simulink model "spring_measurements"  (R2014a)
settings: Solver=FixedStepDiscrete  StartTime=0.0  StopTime=inf  FixedStep=sample_time  RelTol=1e-3
values from neighbouring files (symbols this model uses):
  sample_time = 1/update_freq    (= 0.001)    [init_spring_measurements.m]
undefined symbols (not defined in the file or in its folder): A1_notch_f1, A2_notch_f1, A_lpf_accel, A_lpf_dtau, B1_lpf_accel, B1_lpf_dtau, B1_notch_f1, B2_lpf_accel, B2_lpf_dtau, B2_notch_f1, boom_mount_angle, chirp_amplitude, chirp_bias, chirp_sweep_time, control_start_time, DiscIntNeverNeededParam, ff_motor_position_back, ff_motor_position_front, hip_gravity_compensation, i_limit_lateral, j_segments, k_ff, K_notch_f1, k_sea, kd_lateral, kd_motor_position, kd_motor_velocity, kd_ratio, kd_sea_torque_flight, kd_sea_torque_stance, ki_lateral, kp_lateral, kp_motor_position, kp_motor_velocity, kp_sea_torque_flight, kp_sea_torque_stance, l_seg, lateral_torque_ramp_time, max_sagittal_loaded_torque, max_sagittal_unloaded_torque, max_torque_lateral, sagittal_torque_ramp_time, sawtooth_peak_value, sawtooth_slope, sea_control_torque_cmd_small_threshold, sea_coulomb_friction, sea_extra_moving_friction, sea_offset_friction, sea_static_friction, sine_freq, stance_flight_torque_threshold
libraries: simulink x13, dspsrcs4 x1
settings Model: BufferReuse=off  Creator=wmartin  LastModifiedBy=wmartin
settings SolverCC: EnableConcurrentExecution=on
settings DataIOCC: MaxDataPoints=1000000000  SaveFormat=StructureWithTime
settings OptimizationCC: BlockReduction=off  OptimizeBlockIOStorage=off  BufferReuse=off  GlobalBufferReuse=off  ExpressionFolding=off  ExpressionDepthLimit=2147483647  LocalBlockOutputs=off  SimCompilerOptimization=On
settings DebuggingCC: UnderspecifiedInitializationDetection=Classic  StateNameClashWarn=warning
settings HardwareCC: ProdIntDivRoundTo=Zero  ProdEndianess=LittleEndian  ProdHWDeviceType=Generic->32-bit x86 compatible
settings RTWCC: SystemTargetFile=slrt.tlc  TemplateMakefile=slrt_default_tmf  Description=Simulink Real-Time  RTWVerbose=off  ProcessScript=slrt_make_rtw_hook  RTWCompilerOptimization=On
settings SimulinkRealTimeCC: GeneratePreprocessorConditionals=Disable all  EnableShiftOperators=on  RL32LogBufSizeModifier=100000000

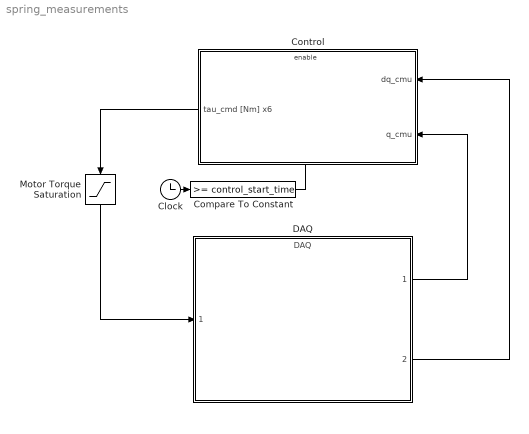
== system spring_measurements ==
  Clock : Clock
  Compare To Constant : simulink/Logic and Bit Operations/Compare To Constant  relop=>=  const=control_start_time  OutDataTypeStr=boolean
  Control : Subsystem
  DAQ : ModelReference  ModelNameDialog=DAQ  SimulationMode=Normal  ModelReferenceVersion=1.1394  CopyOfModelName=DAQ  DefaultDataLogging=on
  Motor Torque Saturation : Saturate  UpperLimit=178.5  LowerLimit=-178.5
      settings: AttributesFormatString=Top: %<UpperLimit>\nBottom: %<LowerLimit>
  wires:
  Clock/1 -> Compare To Constant/1
  Motor Torque Saturation/1 -> DAQ/1
  Compare To Constant/1 -> Control/Enable
  DAQ/1 -> Control/2(q_cmu)
  DAQ/2 -> Control/1(dq_cmu)
  Control/1(tau_cmd [Nm] x6) -> Motor Torque Saturation/1

== system spring_measurements/Control ==
  dq_cmu : Inport
  q_cmu : Inport  Port=2
  Enable : EnablePort  StatesWhenEnabling=reset
  Actuator Control : Subsystem
  Behavior Control : Subsystem
  tau_cmd [Nm] x6 : Outport  InitialOutput=[0 0 0 0 0 0]
  wires:
  q_cmu/1 -> Behavior Control/2(q_cmu), Actuator Control/2(q_cmu)
  dq_cmu/1 -> Behavior Control/1(dq_cmu), Actuator Control/3(dq_cmu)
  Actuator Control/1(tau_cmd [Nm] x6) -> tau_cmd [Nm] x6/1
  Behavior Control/1(motor_torque_cmd) -> Actuator Control/1(tau_desired [Nm] x6)

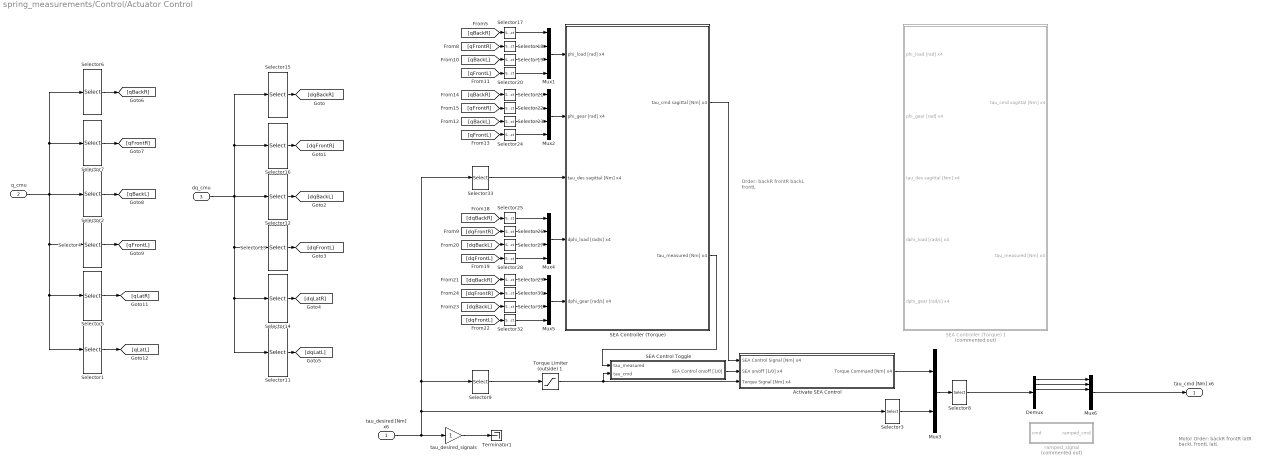
== system spring_measurements/Control/Actuator Control ==
  note: Order:
      | backR
      | frontR
      | backL
      | frontL
  note: Motor Order:
      |
      | backR
      | frontR
      | latR
      | backL
      | frontL
      | latL
  tau_desired [Nm] x6 : Inport
  q_cmu : Inport  Port=2
  dq_cmu : Inport  Port=3
  Activate SEA Control : Subsystem
  Demux : Demux  Outputs=6
  Mux{1..2,4..5} (4 alike) : Mux
  Mux3 : Mux  Inputs=2
  Mux6 : Mux  Inputs=6
  SEA Control Toggle : Subsystem
  SEA Controller (Torque) : Subsystem
  SEA Controller (Torque) 1 : Subsystem  Commented=on
  Selector1 : Selector  InputPortWidth=13  Indices=[10]
  Selector11 : Selector  InputPortWidth=13  Indices=[10]
  Selector12 : Selector  InputPortWidth=13  Indices=[5 6]
  Selector13 : Selector  InputPortWidth=13  Indices=[7 8]
  Selector14 : Selector  InputPortWidth=13  Indices=[9]
  Selector15 : Selector  InputPortWidth=13  Indices=[1 2]
  Selector16 : Selector  InputPortWidth=13  Indices=[3 4]
  Selector{17..20,25..28} (8 alike) : Selector  InputPortWidth=2  Indices=[1]
  Selector2 : Selector  InputPortWidth=13  Indices=[5 6]
  Selector{21..24,29..32} (8 alike) : Selector  InputPortWidth=2  Indices=[2]
  Selector3 : Selector  InputPortWidth=6  Indices=[3 6]
  Selector33 : Selector  InputPortWidth=6  Indices=[1 2 4 5]
  Selector4 : Selector  InputPortWidth=13  Indices=[7 8]
  Selector5 : Selector  InputPortWidth=13  Indices=[9]
  Selector6 : Selector  InputPortWidth=13  Indices=[1 2]
  Selector7 : Selector  InputPortWidth=13  Indices=[3 4]
  Selector8 : Selector  InputPortWidth=6  Indices=[1 2 5 3 4 6]
  Selector9 : Selector  InputPortWidth=6  Indices=[1 2 4 5]
  Terminator1 : Terminator
  Torque Limiter (outside) 1 : Saturate  UpperLimit=max_sagittal_unloaded_torque  LowerLimit=-max_sagittal_unloaded_torque
      settings: AttributesFormatString=Hi: %<UpperLimit>\nLo: %<LowerLimit>
  ramped_signal : Subsystem  Commented=on
  tau_desired_signals : Gain  Description=xPCTag(1)=tau_cmd_signal;
  tau_cmd [Nm] x6 : Outport  InitialOutput=[0 0 0 0 0 0]
  wires:
  Torque Limiter (outside) 1/1 -> SEA Control Toggle/2(tau_cmd), Activate SEA Control/3(Torque Signal [Nm] x4)
  SEA Controller (Torque)/1(tau_cmd sagittal [Nm] x4) -> Activate SEA Control/1(SEA Control Signal [Nm] x4)
  tau_desired [Nm] x6/1 -> tau_desired_signals/1, Selector3/1, Selector33/1, Selector9/1
  Mux6/1 -> tau_cmd [Nm] x6/1
  tau_desired_signals/1 -> Terminator1/1
  Selector5/1 -> [qLatR]
  Selector1/1 -> [qLatL]
  Selector6/1 -> [qBackR]
  Selector7/1 -> [qFrontR]
  Selector2/1 -> [qBackL]
  Selector4/1 -> [qFrontL]
  q_cmu/1 -> Selector1/1, Selector5/1, Selector4/1, Selector6/1, Selector7/1, Selector2/1
  dq_cmu/1 -> Selector12/1, Selector16/1, Selector15/1, Selector13/1, Selector14/1, Selector11/1
  Selector14/1 -> [dqLatR]
  Selector11/1 -> [dqLatL]
  Selector15/1 -> [dqBackR]
  Selector16/1 -> [dqFrontR]
  Selector12/1 -> [dqBackL]
  Selector13/1 -> [dqFrontL]
  Mux1/1 -> SEA Controller (Torque)/1(phi_load [rad] x4)
  [qBackR] -> Selector17/1
  Selector17/1 -> Mux1/1
  Selector19/1 -> Mux1/3
  Selector18/1 -> Mux1/2
  Selector20/1 -> Mux1/4
  [qFrontR] -> Selector18/1
  [qBackL] -> Selector19/1
  [qFrontL] -> Selector20/1
  Mux2/1 -> SEA Controller (Torque)/2(phi_gear [rad] x4)
  [qBackR] -> Selector21/1
  Selector21/1 -> Mux2/1
  Selector23/1 -> Mux2/3
  Selector22/1 -> Mux2/2
  Selector24/1 -> Mux2/4
  [qFrontR] -> Selector22/1
  [qBackL] -> Selector23/1
  [qFrontL] -> Selector24/1
  Mux4/1 -> SEA Controller (Torque)/4(dphi_load [rad/s] x4)
  [dqBackR] -> Selector25/1
  Selector25/1 -> Mux4/1
  Selector27/1 -> Mux4/3
  Selector26/1 -> Mux4/2
  Selector28/1 -> Mux4/4
  [dqFrontR] -> Selector26/1
  [dqBackL] -> Selector27/1
  [dqFrontL] -> Selector28/1
  Mux5/1 -> SEA Controller (Torque)/5(dphi_gear [rad/s] x4)
  [dqBackR] -> Selector29/1
  Selector29/1 -> Mux5/1
  Selector31/1 -> Mux5/3
  Selector30/1 -> Mux5/2
  Selector32/1 -> Mux5/4
  [dqFrontR] -> Selector30/1
  [dqBackL] -> Selector31/1
  [dqFrontL] -> Selector32/1
  Selector33/1 -> SEA Controller (Torque)/3(tau_des sagittal [Nm] x4)
  Selector3/1 -> Mux3/2
  Mux3/1 -> Selector8/1
  Selector8/1 -> Demux/1
  Demux/3 -> Mux6/3
  Demux/1 -> Mux6/1
  Demux/2 -> Mux6/2
  Selector9/1 -> Torque Limiter (outside) 1/1
  SEA Controller (Torque)/2(tau_measured [Nm] x4) -> SEA Control Toggle/1(tau_measured)
  SEA Control Toggle/1(SEA Control on/off [1/0]) -> Activate SEA Control/2("SEA on/off [1/0] x4 ")
  Activate SEA Control/1(Torque Command [Nm] x4) -> Mux3/1

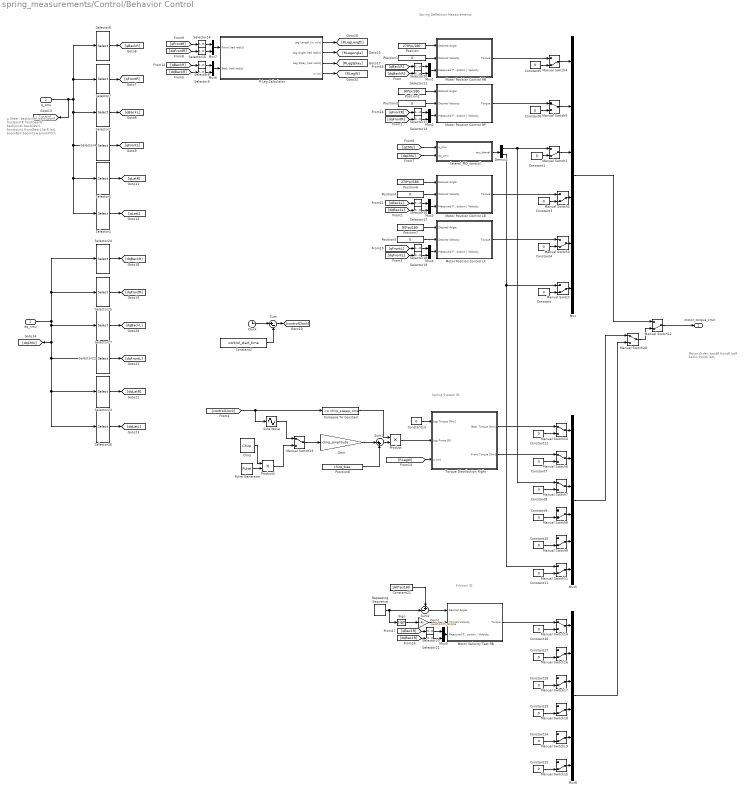
== system spring_measurements/Control/Behavior Control ==
  note: Spring Deflection Measurements
  note: q Order:
      |
      | backJointR
      | backGearR
      | frontJointR
      | frontGearR
      |
      | backJointL
      | backGearL
      | frontJointL
      | frontGearL
      |
      | latR
      | latL
      |
      | boomRoll
      | boomYaw
      | boomPitch
  note: Motor Order:
      |
      | backR
      | frontR
      | latR
      | backL
      | frontL
      | latL
  note: Spring System ID
  note: Friction ID
  dq_cmu : Inport
  q_cmu : Inport  Port=2
  Chirp : dspsrcs4/Chirp  sweep=Quadratic  mode=Unidirectional  f0=chirp_min_freq  f1=chirp_max_freq  t1=chirp_sweep_time  Tsweep=chirp_sweep_time  phase=0  Ts=sample_time  spf=1  datatype=Double
  Clock : Clock
  Compare To Constant : simulink/Logic and Bit Operations/Compare To Constant  relop=<=  const=chirp_sweep_time  OutDataTypeStr=uint8
  Constant{,1,3..19} (19 alike) : Constant  Value=0
  Constant2 : Constant  Value=control_start_time
  Constant21 : Constant  Value=160*pi/180
  Demux2 : Demux  Outputs=2
  Gain : Gain  Gain=chirp_amplitude
  Gain1 : Gain  Gain=-sawtooth_slope
  Manual Switch{,1..4,8..9,11..12,15..19} (14 alike) : ManualSwitch  CurrentSetting=0
  Manual Switch{5..7,10,13..14,20} (7 alike) : ManualSwitch
  Motor Position Control LB : Subsystem
  Motor Position Control LF : Subsystem
  Motor Position Control RB : Subsystem
  Motor Position Control RF : Subsystem
  Motor Velocity Test RB : Subsystem
  Mux : Mux  Inputs=6
  Mux{1..4,6..7,9} (7 alike) : Mux  Inputs=2
  Mux5 : Mux  Inputs=6
  Mux8 : Mux  Inputs=6
  Position : Constant  Value=270*pi/180
  Position{1,3..5} (4 alike) : Constant  Value=0
  Position2 : Constant  Value=90*pi/180
  Position6 : Constant  Value=270*pi/180
  Position7 : Constant  Value=90*pi/180
  Position8 : Constant  Value=chirp_bias
  Product : Product
  Product1 : Product
  Pulse Generator : DiscretePulseGenerator  PulseType=Time based  Period=10  PulseWidth=50
  R Leg Calculator : Subsystem
  Repeating Sequence : simulink/Sources/Repeating Sequence  rep_seq_t=sawtooth_time_values  rep_seq_y=[0 sawtooth_peak_value 0]
  Selector1 : Selector  InputPortWidth=13  Indices=[10]
  Selector{10..13,16..21} (10 alike) : Selector  InputPortWidth=2  Indices=[2]
  Selector{8..9,14..15} (4 alike) : Selector  InputPortWidth=2  Indices=[1]
  Selector2 : Selector  InputPortWidth=13  Indices=[5 6]
  Selector22 : Selector  InputPortWidth=13  Indices=[7 8]
  Selector23 : Selector  InputPortWidth=13  Indices=[9]
  Selector24 : Selector  InputPortWidth=13  Indices=[1 2]
  Selector25 : Selector  InputPortWidth=13  Indices=[3 4]
  Selector26 : Selector  InputPortWidth=13  Indices=[10]
  Selector27 : Selector  InputPortWidth=13  Indices=[5 6]
  Selector4 : Selector  InputPortWidth=13  Indices=[7 8]
  Selector5 : Selector  InputPortWidth=13  Indices=[9]
  Selector6 : Selector  InputPortWidth=13  Indices=[1 2]
  Selector7 : Selector  InputPortWidth=13  Indices=[3 4]
  Sign : Signum
  Sine Wave : Sin  TimeSource=Use external signal  Frequency=sine_freq  SampleTime=0
  Sum : Sum  Inputs=|+-
  Sum1 : Sum  Inputs=|++
  Sum2 : Sum  Inputs=+-|
  Torque Distribution Right : Subsystem
  lateral_PID_control : Subsystem
  motor_torque_cmd : Outport  OutputWhenDisabled=reset  InitialOutput=[0 0 0 0 0 0]
  wires:
  Mux/1 -> Manual Switch12/1
  Demux2/1 -> Manual Switch7/1, Manual Switch1/1
  Demux2/2 -> Manual Switch11/1, Manual Switch/1
  Manual Switch1/1 -> Mux/3
  Manual Switch/1 -> Mux/6
  Constant/1 -> Manual Switch/2
  Constant1/1 -> Manual Switch1/2
  Clock/1 -> Sum/1
  Constant2/1 -> Sum/2
  Selector5/1 -> [qLatR]
  Selector1/1 -> [qLatL]
  Sum/1 -> [controlClock]
  Selector12/1 -> Mux2/1
  Selector16/1 -> Mux3/1
  Selector18/1 -> Mux4/1
  [qCMU] -> lateral_PID_control/1(q_cmu)
  [dqCMU] -> lateral_PID_control/2(dq_cmu)
  lateral_PID_control/1(tau_lateral) -> Demux2/1
  Constant3/1 -> Manual Switch2/2
  Constant4/1 -> Manual Switch3/2
  Manual Switch3/1 -> Mux/5
  Manual Switch2/1 -> Mux/4
  Motor Position Control RB/1(Torque) -> Manual Switch4/1
  Constant5/1 -> Manual Switch4/2
  Constant6/1 -> Manual Switch5/2
  Manual Switch4/1 -> Mux/1
  Manual Switch5/1 -> Mux/2
  Position/1 -> Motor Position Control RB/1(Desired Angle)
  Position1/1 -> Motor Position Control RB/2(Desired Velocity)
  Mux1/1 -> Motor Position Control RB/3(Measured Position / Velocity)
  Selector11/1 -> Mux1/2
  Selector10/1 -> Mux1/1
  Motor Position Control RF/1(Torque) -> Manual Switch5/1
  Mux2/1 -> Motor Position Control RF/3(Measured Position / Velocity)
  Selector13/1 -> Mux2/2
  Position3/1 -> Motor Position Control RF/2(Desired Velocity)
  Position2/1 -> Motor Position Control RF/1(Desired Angle)
  Motor Position Control LB/1(Torque) -> Manual Switch2/1
  Motor Position Control LF/1(Torque) -> Manual Switch3/1
  Mux3/1 -> Motor Position Control LB/3(Measured Position / Velocity)
  Mux4/1 -> Motor Position Control LF/3(Measured Position / Velocity)
  Selector17/1 -> Mux3/2
  Selector19/1 -> Mux4/2
  Position4/1 -> Motor Position Control LB/2(Desired Velocity)
  Position5/1 -> Motor Position Control LF/2(Desired Velocity)
  Position6/1 -> Motor Position Control LB/1(Desired Angle)
  Position7/1 -> Motor Position Control LF/1(Desired Angle)
  Constant12/1 -> Manual Switch10/2
  Constant7/1 -> Manual Switch6/2
  Manual Switch6/1 -> Mux5/2
  Constant8/1 -> Manual Switch7/2
  Manual Switch7/1 -> Mux5/3
  Constant9/1 -> Manual Switch8/2
  Constant10/1 -> Manual Switch9/2
  Constant11/1 -> Manual Switch11/2
  Manual Switch11/1 -> Mux5/6
  Manual Switch9/1 -> Mux5/5
  Manual Switch12/1 -> motor_torque_cmd/1
  Mux5/1 -> Manual Switch20/1
  Manual Switch13/1 -> Gain/1
  [controlClock] -> Sine Wave/1, Compare To Constant/1
  Compare To Constant/1 -> Product/1
  Sum1/1 -> Product/2
  Gain/1 -> Sum1/1
  Position8/1 -> Sum1/2
  Manual Switch10/1 -> Mux5/1
  Manual Switch8/1 -> Mux5/4
  Chirp/1 -> Product1/1
  Sine Wave/1 -> Manual Switch13/1
  Pulse Generator/1 -> Product1/2
  Product1/1 -> Manual Switch13/2
  Product/1 -> Torque Distribution Right/2(Leg Force [N])
  Torque Distribution Right/1(Back Torque [Nm]) -> Manual Switch10/1
  Torque Distribution Right/2(Front Torque [Nm]) -> Manual Switch6/1
  Constant13/1 -> Torque Distribution Right/1(Leg Torque [Nm])
  Mux7/1 -> R Leg Calculator/1(Front [rad rad/s])
  Mux6/1 -> R Leg Calculator/2(Back [rad rad/s])
  R Leg Calculator/1("Leg Length [m m/s] ") -> [RLegLength]
  R Leg Calculator/2(Leg Angle [rad rad/s]) -> [RLegAngle]
  R Leg Calculator/3(Leg Splay [rad rad/s]) -> [RLegSplay]
  Selector14/1 -> Mux7/1
  Selector15/1 -> Mux7/2
  Selector9/1 -> Mux6/2
  Selector8/1 -> Mux6/1
  R Leg Calculator/4(w [m]) -> [RLegW]
  [RLegW] -> Torque Distribution Right/3(w [m])
  Constant16/1 -> Manual Switch14/2
  Constant17/1 -> Manual Switch16/2
  Manual Switch16/1 -> Mux8/2
  Constant18/1 -> Manual Switch17/2
  Manual Switch17/1 -> Mux8/3
  Constant19/1 -> Manual Switch18/2
  Constant14/1 -> Manual Switch19/2
  Constant15/1 -> Manual Switch15/2
  Manual Switch15/1 -> Mux8/6
  Manual Switch19/1 -> Mux8/5
  Mux8/1 -> Manual Switch20/2
  Manual Switch14/1 -> Mux8/1
  Manual Switch18/1 -> Mux8/4
  Motor Velocity Test RB/1(Torque) -> Manual Switch14/1
  q_cmu/1 -> [qCMU], Selector6/1, Selector7/1, Selector2/1, Selector4/1, Selector1/1, Selector5/1
  Selector4/1 -> [qFrontL]
  Selector2/1 -> [qBackL]
  Selector7/1 -> [qFrontR]
  Selector6/1 -> [qBackR]
  [dqBackR] -> Selector9/1
  [qBackR] -> Selector8/1
  [dqFrontR] -> Selector15/1
  [qFrontR] -> Selector14/1
  [qBackR] -> Selector10/1
  [dqBackR] -> Selector11/1
  [qFrontR] -> Selector12/1
  [dqFrontR] -> Selector13/1
  [qFrontL] -> Selector18/1
  [dqFrontL] -> Selector19/1
  [dqBackL] -> Selector17/1
  [qBackL] -> Selector16/1
  [qBackR] -> Selector20/1
  [dqBackR] -> Selector21/1
  Selector26/1 -> [dqLatL]
  Selector23/1 -> [dqLatR]
  Selector24/1 -> [dqBackR]
  Selector25/1 -> [dqFrontR]
  Selector27/1 -> [dqBackL]
  Selector22/1 -> [dqFrontL]
  dq_cmu/1 -> Selector27/1, Selector26/1, Selector23/1, Selector22/1, [dqCMU], Selector24/1, Selector25/1
  Repeating Sequence/1 -> Sign/1, Sum2/2
  Mux9/1 -> Motor Velocity Test RB/3(Measured Position / Velocity)
  Selector21/1 -> Mux9/2
  Selector20/1 -> Mux9/1
  Sign/1 -> Gain1/1
  Gain1/1 -> Motor Velocity Test RB/2(Desired Velocity)
  Sum2/1 -> Motor Velocity Test RB/1(Desired Angle)
  Constant21/1 -> Sum2/1
  Manual Switch20/1 -> Manual Switch12/2

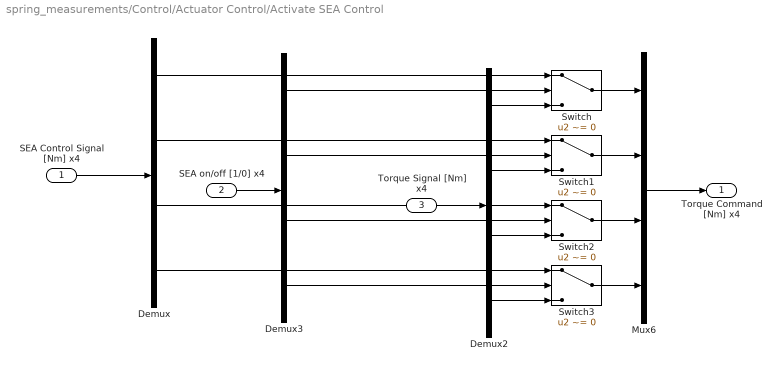
== system spring_measurements/Control/Actuator Control/Activate SEA Control ==
  SEA Control Signal [Nm] x4 : Inport
  "SEA on/off [1/0] x4 " : Inport  Port=2
  Torque Signal [Nm] x4 : Inport  Port=3
  Demux : Demux
  Demux2 : Demux
  Demux3 : Demux
  Mux6 : Mux
  Switch{,1..3} (4 alike) : Switch  Criteria=u2 ~= 0
  Torque Command [Nm] x4 : Outport
  wires:
  Torque Signal [Nm] x4/1 -> Demux2/1
  "SEA on/off [1/0] x4 "/1 -> Demux3/1
  SEA Control Signal [Nm] x4/1 -> Demux/1
  Demux2/3 -> Switch2/3
  Demux/2 -> Switch1/1
  Demux3/4 -> Switch3/2
  Demux2/4 -> Switch3/3
  Demux/4 -> Switch3/1
  Switch2/1 -> Mux6/3
  Demux/3 -> Switch2/1
  Demux3/2 -> Switch1/2
  Demux3/3 -> Switch2/2
  Mux6/1 -> Torque Command [Nm] x4/1
  Demux3/1 -> Switch/2
  Switch3/1 -> Mux6/4
  Switch1/1 -> Mux6/2
  Switch/1 -> Mux6/1
  Demux/1 -> Switch/1
  Demux2/1 -> Switch/3
  Demux2/2 -> Switch1/3

== system spring_measurements/Control/Actuator Control/SEA Control Toggle ==
  tau_measured : Inport
  tau_cmd : Inport  Port=2
  Abs : Abs
  Abs1 : Abs
  But Commanding a Small Torque? : simulink/Logic and Bit Operations/Compare To Constant  relop=<  const=sea_control_torque_cmd_small_threshold  OutDataTypeStr=boolean
  Logical Operator1 : Logic  AllPortsSameDT=off  OutDataTypeStr=boolean
  Logical Operator2 : Logic  Operator=NOT  AllPortsSameDT=off  OutDataTypeStr=boolean
  Measuring a Large Torque? (High Gains) : simulink/Logic and Bit Operations/Compare To Constant  relop=>=  const=stance_flight_torque_threshold  OutDataTypeStr=boolean
  SEA Control on/off [1/0] : Outport
  wires:
  Abs1/1 -> Measuring a Large Torque? (High Gains)/1
  Measuring a Large Torque? (High Gains)/1 -> Logical Operator1/1
  tau_measured/1 -> Abs1/1
  Abs/1 -> But Commanding a Small Torque?/1
  tau_cmd/1 -> Abs/1
  Logical Operator1/1 -> Logical Operator2/1
  But Commanding a Small Torque?/1 -> Logical Operator1/2
  Logical Operator2/1 -> SEA Control on/off [1/0]/1

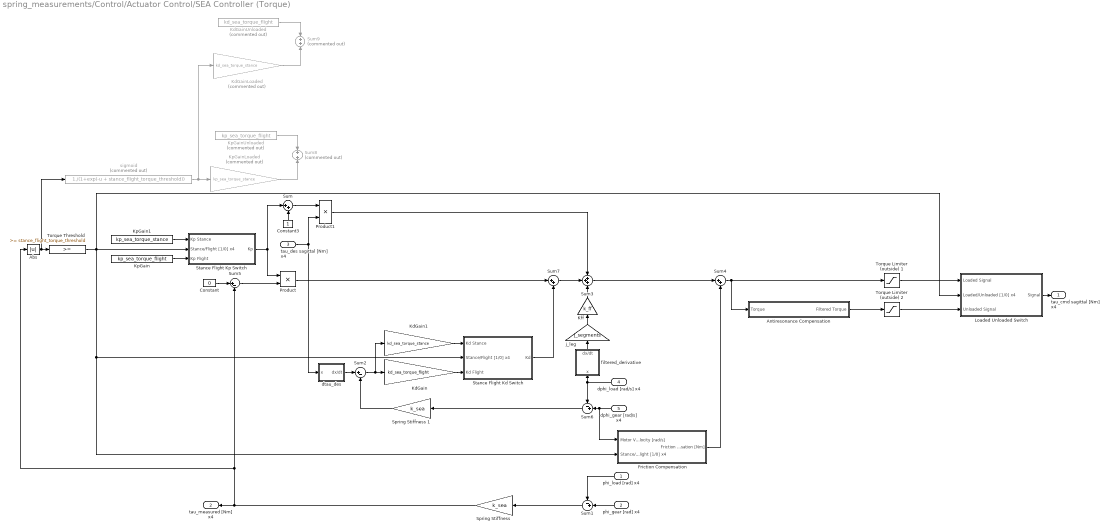
== system spring_measurements/Control/Actuator Control/SEA Controller (Torque) ==
  phi_load [rad] x4 : Inport
  phi_gear [rad] x4 : Inport  Port=2
  tau_des sagittal [Nm] x4 : Inport  Port=3
  dphi_load [rad/s] x4 : Inport  Port=4
  dphi_gear [rad/s] x4 : Inport  Port=5
  Abs : Abs
  Antiresonance Compensation : Subsystem
  Constant : Constant  Value=0
  Constant3 : Constant
  Friction Compensation : Subsystem
  KdGain : Gain  Description=xPCTag(1)=kd_sea_torque;  Gain=kd_sea_torque_flight
  KdGain1 : Gain  Description=xPCTag(1)=kd_sea_torque;  Gain=kd_sea_torque_stance
  KdGainLoaded : Gain  Description=xPCTag(1)=kd_sea_torque;  Commented=on  Gain=kd_sea_torque_stance
  KdGainUnloaded : Constant  Commented=on  Value=kd_sea_torque_flight  SampleTime=sample_time
  Kff : Gain  Gain=k_ff
  KpGain : Constant  Value=kp_sea_torque_flight  SampleTime=sample_time
  KpGain1 : Constant  Value=kp_sea_torque_stance  SampleTime=sample_time
  KpGainLoaded : Gain  Description=xPCTag(1)=kd_sea_torque;  Commented=on  Gain=kp_sea_torque_stance
  KpGainUnloaded : Constant  Commented=on  Value=kp_sea_torque_flight  SampleTime=sample_time
  Loaded Unloaded Switch : Subsystem
  Product : Product  SampleTime=sample_time  RndMeth=Zero
  Product1 : Product  RndMeth=Zero
  Spring Stiffness : Gain  Gain=k_sea
  Spring Stiffness 1 : Gain  Gain=k_sea
  Stance Flight Kd Switch : Subsystem
  Stance Flight Kp Switch : Subsystem
  Sum : Sum  Inputs=|++  SampleTime=sample_time
  Sum1 : Sum  Inputs=-+|
  Sum2 : Sum  Inputs=|+-
  Sum3 : Sum  Inputs=+++
  Sum4 : Sum  Inputs=|++
  Sum5 : Sum  Inputs=|+-
  Sum6 : Sum  Inputs=-+|
  Sum7 : Sum  Inputs=|++
  Sum8 : Sum  Commented=on  Inputs=+|+  SampleTime=sample_time
  Sum9 : Sum  Commented=on  Inputs=+|+  SampleTime=sample_time
  Torque Limiter (outside) 1 : Saturate  UpperLimit=max_sagittal_loaded_torque  LowerLimit=-max_sagittal_loaded_torque
      settings: AttributesFormatString=Hi: %<UpperLimit>\nLo: %<LowerLimit>
  Torque Limiter (outside) 2 : Saturate  UpperLimit=max_sagittal_unloaded_torque  LowerLimit=-max_sagittal_unloaded_torque
      settings: AttributesFormatString=Hi: %<UpperLimit>\nLo: %<LowerLimit>
  Torque Threshold : simulink/Logic and Bit Operations/Compare To Constant  relop=>=  const=stance_flight_torque_threshold  OutDataTypeStr=boolean
  dtau_des : Subsystem
  filtered_derivative : Subsystem
  j_leg : Gain  Description=xPCTag(1)=kd_sea_torque;  Gain=j_segments
  sigmoid : Fcn  Commented=on  Expr=1./(1+exp(-u + stance_flight_torque_threshold))
  tau_cmd sagittal [Nm] x4 : Outport
  tau_measured [Nm] x4 : Outport  Port=2
  wires:
  KdGainLoaded/1 -> Sum9/2
  KdGainUnloaded/1 -> Sum9/1
  KpGainLoaded/1 -> Sum8/2
  KpGainUnloaded/1 -> Sum8/1
  sigmoid/1 -> KpGainLoaded/1, KdGainLoaded/1
  Loaded Unloaded Switch/1(Signal) -> tau_cmd sagittal [Nm] x4/1
  Torque Limiter (outside) 2/1 -> Loaded Unloaded Switch/3(Unloaded Signal)
  Friction Compensation/1(Friction Compensation [Nm]) -> Sum4/2
  tau_des sagittal [Nm] x4/1 -> Product1/2, dtau_des/1(x)
  Kff/1 -> Sum3/3
  Torque Limiter (outside) 1/1 -> Loaded Unloaded Switch/1(Loaded Signal)
  j_leg/1 -> Kff/1
  filtered_derivative/1(dx/dt) -> j_leg/1
  Sum/1 -> Product1/1
  Constant3/1 -> Sum/2
  KdGain/1 -> Stance Flight Kd Switch/3(Kd Flight)
  Product/1 -> Sum7/1
  Sum5/1 -> Product/2
  Sum2/1 -> KdGain1/1, KdGain/1
  dphi_gear [rad/s] x4/1 -> Friction Compensation/1(Motor Velocity [rad/s]), Sum6/2
  dphi_load [rad/s] x4/1 -> filtered_derivative/1(x), Sum6/1
  Spring Stiffness 1/1 -> Sum2/2
  Sum6/1 -> Spring Stiffness 1/1
  dtau_des/1(dx/dt) -> Sum2/1
  Constant/1 -> Sum5/1
  phi_gear [rad] x4/1 -> Sum1/2
  phi_load [rad] x4/1 -> Sum1/1
  Sum1/1 -> Spring Stiffness/1
  KpGain1/1 -> Stance Flight Kp Switch/1(Kp Stance)
  Torque Threshold/1 -> Friction Compensation/2(Stance/Flight [1/0] x4), Stance Flight Kd Switch/2(Stance/Flight [1/0] x4), Stance Flight Kp Switch/2(Stance/Flight [1/0] x4), Loaded Unloaded Switch/2(Loaded/Unloaded [1/0] x4)
  KpGain/1 -> Stance Flight Kp Switch/3(Kp Flight)
  KdGain1/1 -> Stance Flight Kd Switch/1(Kd Stance)
  Spring Stiffness/1 -> Sum5/2, Abs/1, tau_measured [Nm] x4/1
  Stance Flight Kp Switch/1(Kp) -> Sum/1, Product/1
  Abs/1 -> Torque Threshold/1, sigmoid/1
  Stance Flight Kd Switch/1(Kd) -> Sum7/2
  Sum4/1 -> Torque Limiter (outside) 1/1, Antiresonance Compensation/1(Torque)
  Product1/1 -> Sum3/1
  Sum7/1 -> Sum3/2
  Sum3/1 -> Sum4/1
  Antiresonance Compensation/1(Filtered Torque) -> Torque Limiter (outside) 2/1

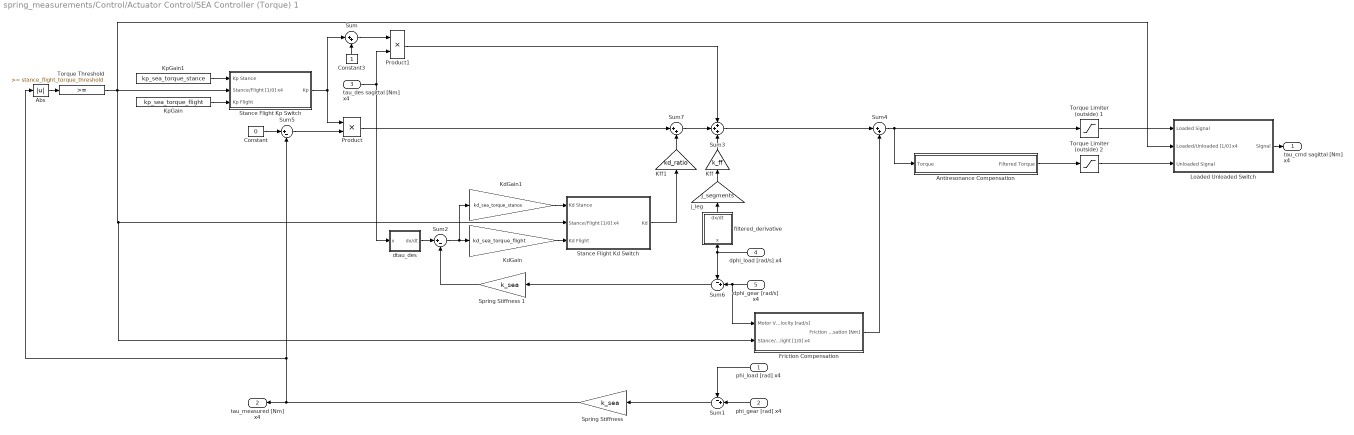
== system spring_measurements/Control/Actuator Control/SEA Controller (Torque) 1 ==
  phi_load [rad] x4 : Inport
  phi_gear [rad] x4 : Inport  Port=2
  tau_des sagittal [Nm] x4 : Inport  Port=3
  dphi_load [rad/s] x4 : Inport  Port=4
  dphi_gear [rad/s] x4 : Inport  Port=5
  Abs : Abs
  Antiresonance Compensation : Subsystem
  Constant : Constant  Value=0
  Constant3 : Constant
  Friction Compensation : Subsystem
  KdGain : Gain  Description=xPCTag(1)=kd_sea_torque;  Gain=kd_sea_torque_flight
  KdGain1 : Gain  Description=xPCTag(1)=kd_sea_torque;  Gain=kd_sea_torque_stance
  Kff : Gain  Gain=k_ff
  Kff1 : Gain  Gain=kd_ratio
  KpGain : Constant  Value=kp_sea_torque_flight  SampleTime=sample_time
  KpGain1 : Constant  Value=kp_sea_torque_stance  SampleTime=sample_time
  Loaded Unloaded Switch : Subsystem
  Product : Product  SampleTime=sample_time  RndMeth=Zero
  Product1 : Product  RndMeth=Zero
  Spring Stiffness : Gain  Gain=k_sea
  Spring Stiffness 1 : Gain  Gain=k_sea
  Stance Flight Kd Switch : Subsystem
  Stance Flight Kp Switch : Subsystem
  Sum : Sum  Inputs=|++  SampleTime=sample_time
  Sum1 : Sum  Inputs=-+|
  Sum2 : Sum  Inputs=|+-
  Sum3 : Sum  Inputs=+++
  Sum4 : Sum  Inputs=|++
  Sum5 : Sum  Inputs=|+-
  Sum6 : Sum  Inputs=-+|
  Sum7 : Sum  Inputs=|++
  Torque Limiter (outside) 1 : Saturate  UpperLimit=max_sagittal_loaded_torque  LowerLimit=-max_sagittal_loaded_torque
      settings: AttributesFormatString=Hi: %<UpperLimit>\nLo: %<LowerLimit>
  Torque Limiter (outside) 2 : Saturate  UpperLimit=max_sagittal_unloaded_torque  LowerLimit=-max_sagittal_unloaded_torque
      settings: AttributesFormatString=Hi: %<UpperLimit>\nLo: %<LowerLimit>
  Torque Threshold : simulink/Logic and Bit Operations/Compare To Constant  relop=>=  const=stance_flight_torque_threshold  OutDataTypeStr=boolean
  dtau_des : Subsystem
  filtered_derivative : Subsystem
  j_leg : Gain  Description=xPCTag(1)=kd_sea_torque;  Gain=j_segments
  tau_cmd sagittal [Nm] x4 : Outport
  tau_measured [Nm] x4 : Outport  Port=2
  wires:
  Loaded Unloaded Switch/1(Signal) -> tau_cmd sagittal [Nm] x4/1
  Torque Limiter (outside) 2/1 -> Loaded Unloaded Switch/3(Unloaded Signal)
  Friction Compensation/1(Friction Compensation [Nm]) -> Sum4/2
  tau_des sagittal [Nm] x4/1 -> Product1/2, dtau_des/1(x)
  Stance Flight Kd Switch/1(Kd) -> Kff1/1
  Kff/1 -> Sum3/3
  Torque Limiter (outside) 1/1 -> Loaded Unloaded Switch/1(Loaded Signal)
  j_leg/1 -> Kff/1
  filtered_derivative/1(dx/dt) -> j_leg/1
  Sum/1 -> Product1/1
  Constant3/1 -> Sum/2
  KdGain/1 -> Stance Flight Kd Switch/3(Kd Flight)
  Product/1 -> Sum7/1
  Sum5/1 -> Product/2
  Sum2/1 -> KdGain1/1, KdGain/1
  dphi_gear [rad/s] x4/1 -> Friction Compensation/1(Motor Velocity [rad/s]), Sum6/2
  dphi_load [rad/s] x4/1 -> filtered_derivative/1(x), Sum6/1
  Spring Stiffness 1/1 -> Sum2/2
  Sum6/1 -> Spring Stiffness 1/1
  dtau_des/1(dx/dt) -> Sum2/1
  Constant/1 -> Sum5/1
  phi_gear [rad] x4/1 -> Sum1/2
  phi_load [rad] x4/1 -> Sum1/1
  Sum1/1 -> Spring Stiffness/1
  KpGain1/1 -> Stance Flight Kp Switch/1(Kp Stance)
  Torque Threshold/1 -> Friction Compensation/2(Stance/Flight [1/0] x4), Stance Flight Kd Switch/2(Stance/Flight [1/0] x4), Stance Flight Kp Switch/2(Stance/Flight [1/0] x4), Loaded Unloaded Switch/2(Loaded/Unloaded [1/0] x4)
  KpGain/1 -> Stance Flight Kp Switch/3(Kp Flight)
  KdGain1/1 -> Stance Flight Kd Switch/1(Kd Stance)
  Spring Stiffness/1 -> Sum5/2, Abs/1, tau_measured [Nm] x4/1
  Stance Flight Kp Switch/1(Kp) -> Sum/1, Product/1
  Abs/1 -> Torque Threshold/1
  Kff1/1 -> Sum7/2
  Sum4/1 -> Torque Limiter (outside) 1/1, Antiresonance Compensation/1(Torque)
  Product1/1 -> Sum3/1
  Sum7/1 -> Sum3/2
  Sum3/1 -> Sum4/1
  Antiresonance Compensation/1(Filtered Torque) -> Torque Limiter (outside) 2/1

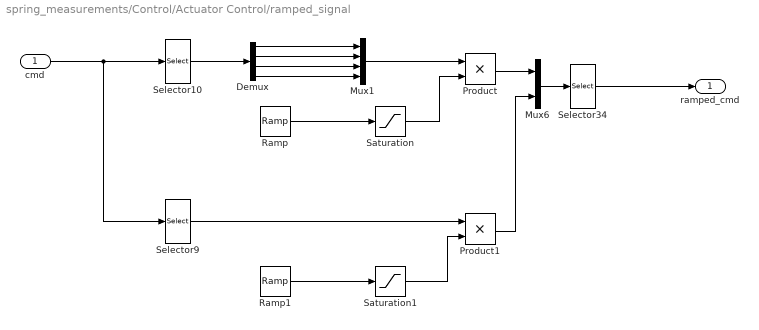
== system spring_measurements/Control/Actuator Control/ramped_signal ==
  cmd : Inport
  Demux : Demux
  Mux1 : Mux
  Mux6 : Mux  Inputs=2
  Product : Product  RndMeth=Zero
  Product1 : Product  RndMeth=Zero
  Ramp : simulink/Sources/Ramp  slope=1/sagittal_torque_ramp_time  start=sagittal_starting_time  X0=0
      settings: AttributesFormatString=Start: %<start>\nSlope: %<slope>
  Ramp1 : simulink/Sources/Ramp  slope=1/lateral_torque_ramp_time  start=control_start_time  X0=0
      settings: AttributesFormatString=Start: %<start>\nSlope: %<slope>
  Saturation : Saturate  UpperLimit=1  LowerLimit=0
      settings: AttributesFormatString=Hi: %<UpperLimit>\nLo: %<LowerLimit>
  Saturation1 : Saturate  UpperLimit=1  LowerLimit=0
      settings: AttributesFormatString=Hi: %<UpperLimit>\nLo: %<LowerLimit>
  Selector10 : Selector  InputPortWidth=6  Indices=[1 2 4 5]
  Selector34 : Selector  InputPortWidth=6  Indices=[1 2 5 3 4 6]
  Selector9 : Selector  InputPortWidth=6  Indices=[3 6]
  ramped_cmd : Outport
  wires:
  Demux/3 -> Mux1/3
  Demux/4 -> Mux1/4
  Mux1/1 -> Product/1
  Demux/2 -> Mux1/2
  Demux/1 -> Mux1/1
  Mux6/1 -> Selector34/1
  Selector10/1 -> Demux/1
  Selector34/1 -> ramped_cmd/1
  Product1/1 -> Mux6/2
  cmd/1 -> Selector9/1, Selector10/1
  Product/1 -> Mux6/1
  Ramp/1 -> Saturation/1
  Saturation/1 -> Product/2
  Ramp1/1 -> Saturation1/1
  Saturation1/1 -> Product1/2
  Selector9/1 -> Product1/1

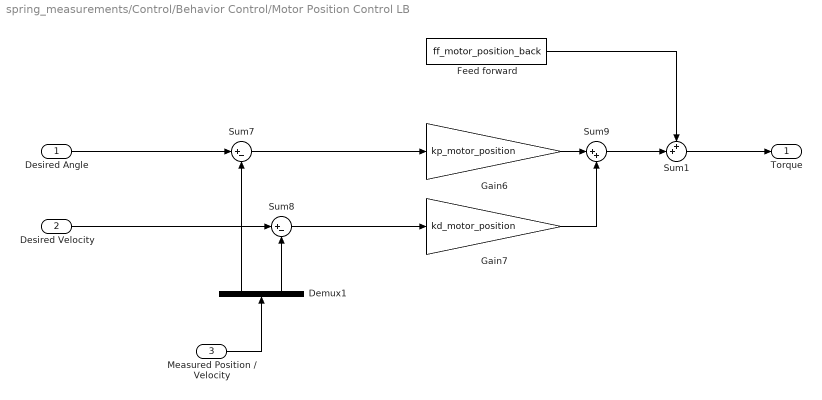
== system spring_measurements/Control/Behavior Control/Motor Position Control LB ==
  Desired Angle : Inport
  Desired Velocity : Inport  Port=2
  Measured Position / Velocity : Inport  Port=3
  Demux1 : Demux  Outputs=2
  Feed forward : Constant  Value=ff_motor_position_back
  Gain6 : Gain  Gain=kp_motor_position
  Gain7 : Gain  Gain=kd_motor_position
  Sum1 : Sum  Inputs=++|
  Sum7 : Sum  Inputs=|+-
  Sum8 : Sum  Inputs=|+-
  Sum9 : Sum  Inputs=|++
  Torque : Outport
  wires:
  Sum7/1 -> Gain6/1
  Demux1/1 -> Sum7/2
  Sum9/1 -> Sum1/2
  Desired Velocity/1 -> Sum8/1
  Sum8/1 -> Gain7/1
  Desired Angle/1 -> Sum7/1
  Demux1/2 -> Sum8/2
  Measured Position / Velocity/1 -> Demux1/1
  Gain7/1 -> Sum9/2
  Gain6/1 -> Sum9/1
  Feed forward/1 -> Sum1/1
  Sum1/1 -> Torque/1

== system spring_measurements/Control/Behavior Control/Motor Position Control LF ==
  Desired Angle : Inport
  Desired Velocity : Inport  Port=2
  Measured Position / Velocity : Inport  Port=3
  Demux1 : Demux  Outputs=2
  Feed forward : Constant  Value=ff_motor_position_front
  Gain6 : Gain  Gain=kp_motor_position
  Gain7 : Gain  Gain=kd_motor_position
  Sum1 : Sum  Inputs=++|
  Sum7 : Sum  Inputs=|+-
  Sum8 : Sum  Inputs=|+-
  Sum9 : Sum  Inputs=|++
  Torque : Outport
  wires:
  Sum1/1 -> Torque/1
  Feed forward/1 -> Sum1/1
  Gain6/1 -> Sum9/1
  Gain7/1 -> Sum9/2
  Measured Position / Velocity/1 -> Demux1/1
  Demux1/2 -> Sum8/2
  Desired Angle/1 -> Sum7/1
  Sum8/1 -> Gain7/1
  Desired Velocity/1 -> Sum8/1
  Sum9/1 -> Sum1/2
  Demux1/1 -> Sum7/2
  Sum7/1 -> Gain6/1

== system spring_measurements/Control/Behavior Control/Motor Position Control RB ==
  Desired Angle : Inport
  Desired Velocity : Inport  Port=2
  Measured Position / Velocity : Inport  Port=3
  Demux1 : Demux  Outputs=2
  Feed forward : Constant  Value=ff_motor_position_back
  Gain6 : Gain  Gain=kp_motor_position
  Gain7 : Gain  Gain=kd_motor_position
  Sum1 : Sum  Inputs=++|
  Sum7 : Sum  Inputs=|+-
  Sum8 : Sum  Inputs=|+-
  Sum9 : Sum  Inputs=|++
  Torque : Outport
  wires:
  Sum7/1 -> Gain6/1
  Demux1/1 -> Sum7/2
  Sum9/1 -> Sum1/2
  Desired Velocity/1 -> Sum8/1
  Sum8/1 -> Gain7/1
  Desired Angle/1 -> Sum7/1
  Demux1/2 -> Sum8/2
  Measured Position / Velocity/1 -> Demux1/1
  Gain7/1 -> Sum9/2
  Gain6/1 -> Sum9/1
  Feed forward/1 -> Sum1/1
  Sum1/1 -> Torque/1

== system spring_measurements/Control/Behavior Control/Motor Position Control RF ==
  Desired Angle : Inport
  Desired Velocity : Inport  Port=2
  Measured Position / Velocity : Inport  Port=3
  Demux1 : Demux  Outputs=2
  Feed forward : Constant  Value=ff_motor_position_front
  Gain6 : Gain  Gain=kp_motor_position
  Gain7 : Gain  Gain=kd_motor_position
  Sum1 : Sum  Inputs=++|
  Sum7 : Sum  Inputs=|+-
  Sum8 : Sum  Inputs=|+-
  Sum9 : Sum  Inputs=|++
  Torque : Outport
  wires:
  Sum1/1 -> Torque/1
  Feed forward/1 -> Sum1/1
  Gain6/1 -> Sum9/1
  Gain7/1 -> Sum9/2
  Measured Position / Velocity/1 -> Demux1/1
  Demux1/2 -> Sum8/2
  Desired Angle/1 -> Sum7/1
  Sum8/1 -> Gain7/1
  Desired Velocity/1 -> Sum8/1
  Sum9/1 -> Sum1/2
  Demux1/1 -> Sum7/2
  Sum7/1 -> Gain6/1

== system spring_measurements/Control/Behavior Control/Motor Velocity Test RB ==
  Desired Angle : Inport
  Desired Velocity : Inport  Port=2
  Measured Position / Velocity : Inport  Port=3
  Demux1 : Demux  Outputs=2
  Gain6 : Gain  Gain=kp_motor_velocity
  Gain7 : Gain  Gain=kd_motor_velocity
  Sum7 : Sum  Inputs=|+-
  Sum8 : Sum  Inputs=|+-
  Sum9 : Sum  Inputs=|++
  Torque : Outport
  wires:
  Sum9/1 -> Torque/1
  Gain6/1 -> Sum9/1
  Gain7/1 -> Sum9/2
  Measured Position / Velocity/1 -> Demux1/1
  Demux1/2 -> Sum8/2
  Desired Angle/1 -> Sum7/1
  Sum8/1 -> Gain7/1
  Desired Velocity/1 -> Sum8/1
  Demux1/1 -> Sum7/2
  Sum7/1 -> Gain6/1

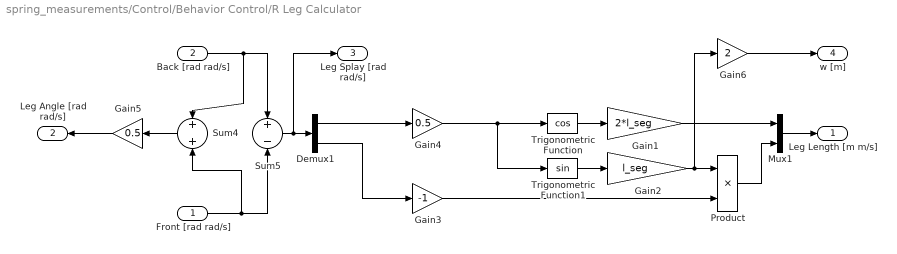
== system spring_measurements/Control/Behavior Control/R Leg Calculator ==
  Front [rad rad/s] : Inport
  Back [rad rad/s] : Inport  Port=2
  Demux1 : Demux  Outputs=2
  Gain1 : Gain  Gain=2*l_seg
  Gain2 : Gain  Gain=l_seg
  Gain3 : Gain  Gain=-1
  Gain4 : Gain  Gain=0.5
  Gain5 : Gain  Gain=0.5
  Gain6 : Gain  Gain=2
  Mux1 : Mux  Inputs=2
  Product : Product  RndMeth=Zero
  Sum4 : Sum  Inputs=+|+
  Sum5 : Sum  Inputs=+|-
  Trigonometric Function : Trigonometry  Operator=cos
  Trigonometric Function1 : Trigonometry
  "Leg Length [m m/s] " : Outport
  Leg Angle [rad rad/s] : Outport  Port=2
  Leg Splay [rad rad/s] : Outport  Port=3
  w [m] : Outport  Port=4
  wires:
  Gain5/1 -> Leg Angle [rad rad/s]/1
  Sum4/1 -> Gain5/1
  Mux1/1 -> "Leg Length [m m/s] "/1
  Sum5/1 -> Demux1/1, Leg Splay [rad rad/s]/1
  Gain2/1 -> Gain6/1, Product/1
  Demux1/1 -> Gain4/1
  Gain3/1 -> Product/2
  Demux1/2 -> Gain3/1
  Back [rad rad/s]/1 -> Sum5/1, Sum4/1
  Front [rad rad/s]/1 -> Sum4/2, Sum5/2
  Product/1 -> Mux1/2
  Trigonometric Function1/1 -> Gain2/1
  Gain1/1 -> Mux1/1
  Trigonometric Function/1 -> Gain1/1
  Gain4/1 -> Trigonometric Function/1, Trigonometric Function1/1
  Gain6/1 -> w [m]/1

== system spring_measurements/Control/Behavior Control/Torque Distribution Right ==
  Leg Torque [Nm] : Inport
  Leg Force [N] : Inport  Port=2
  w [m] : Inport  Port=3
  Gain : Gain  Gain=0.5
  Gain1 : Gain  Gain=0.5
  Product : Product  RndMeth=Zero
  Sum : Sum  Inputs=|++
  Sum1 : Sum  Inputs=+-|
  Back Torque [Nm] : Outport
  Front Torque [Nm] : Outport  Port=2
  wires:
  Product/1 -> Gain1/1
  Leg Force [N]/1 -> Product/1
  Gain1/1 -> Sum/2, Sum1/2
  w [m]/1 -> Product/2
  Gain/1 -> Sum1/1, Sum/1
  Sum/1 -> Front Torque [Nm]/1
  Leg Torque [Nm]/1 -> Gain/1
  Sum1/1 -> Back Torque [Nm]/1

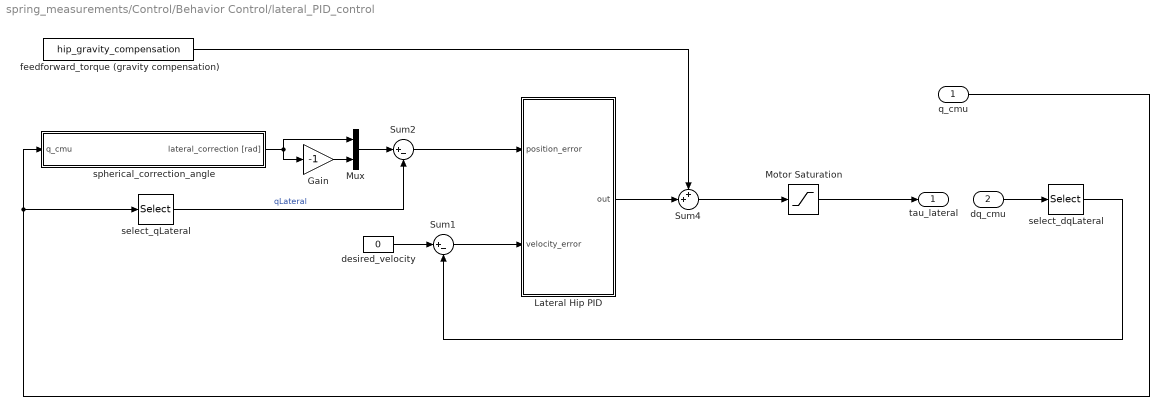
== system spring_measurements/Control/Behavior Control/lateral_PID_control ==
  q_cmu : Inport
  dq_cmu : Inport  Port=2
  Gain : Gain  Gain=-1
  Lateral Hip PID : Subsystem
  Motor Saturation : Saturate  UpperLimit=max_torque_lateral  LowerLimit=-max_torque_lateral
      settings: AttributesFormatString=Top: %<UpperLimit>\nBottom: %<LowerLimit>
  Mux : Mux  Inputs=2
  Sum1 : Sum  Inputs=|+-
  Sum2 : Sum  Inputs=|+-
  Sum4 : Sum  Inputs=++|
  desired_velocity : Constant  Value=0
  feedforward_torque (gravity compensation) : Constant  Value=hip_gravity_compensation
  select_dqLateral : Selector  InputPortWidth=13  Indices=[9 10]
  select_qLateral : Selector  InputPortWidth=13  Indices=[9 10]
  spherical_correction_angle : Subsystem
  tau_lateral : Outport
  wires:
  Motor Saturation/1 -> tau_lateral/1
  select_qLateral/1 -> Sum2/2  "qLateral"
  Mux/1 -> Sum2/1
  Gain/1 -> Mux/2
  feedforward_torque (gravity compensation)/1 -> Sum4/1
  Sum1/1 -> Lateral Hip PID/2(velocity_error)
  desired_velocity/1 -> Sum1/1
  Sum4/1 -> Motor Saturation/1
  dq_cmu/1 -> select_dqLateral/1
  select_dqLateral/1 -> Sum1/2
  q_cmu/1 -> select_qLateral/1, spherical_correction_angle/1(q_cmu)
  Sum2/1 -> Lateral Hip PID/1(position_error)
  Lateral Hip PID/1(out) -> Sum4/2
  spherical_correction_angle/1(lateral_correction [rad]) -> Gain/1, Mux/1

== system spring_measurements/Control/Actuator Control/SEA Controller (Torque)/Antiresonance Compensation ==
  Torque : Inport
  Notch Filter (Flight) : DiscreteTransferFcn  Numerator=[K_notch_f1 K_notch_f1*A1_notch_f1 K_notch_f1*A2_notch_f1]  Denominator=[1 B1_notch_f1 B2_notch_f1]  SampleTime=sample_time
  Filtered Torque : Outport
  wires:
  Notch Filter (Flight)/1 -> Filtered Torque/1
  Torque/1 -> Notch Filter (Flight)/1

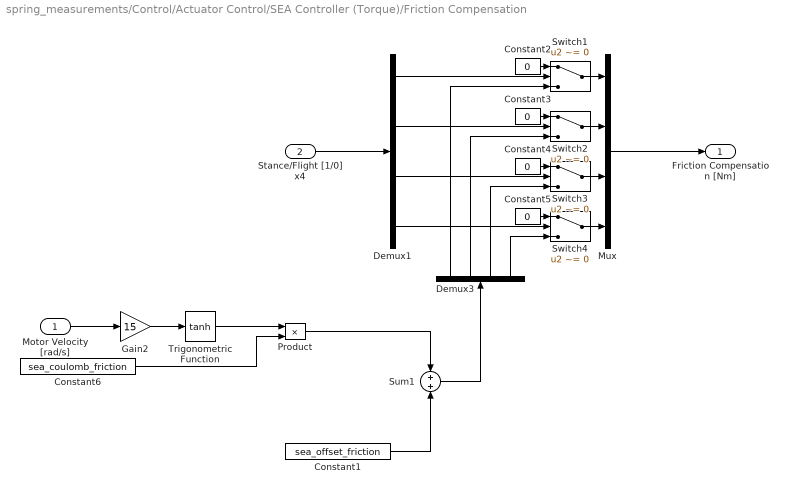
== system spring_measurements/Control/Actuator Control/SEA Controller (Torque)/Friction Compensation ==
  Motor Velocity [rad/s] : Inport
  Stance/Flight [1/0] x4 : Inport  Port=2
  Constant1 : Constant  Value=sea_offset_friction
  Constant{2..5} (4 alike) : Constant  Value=0
  Constant6 : Constant  Value=sea_coulomb_friction
  Demux1 : Demux
  Demux3 : Demux
  Gain2 : Gain  Gain=15
  Mux : Mux
  Product : Product
  Sum1 : Sum
  Switch{1..4} (4 alike) : Switch  Criteria=u2 ~= 0
  Trigonometric Function : Trigonometry  Operator=tanh
  Friction Compensation [Nm] : Outport
  wires:
  Mux/1 -> Friction Compensation [Nm]/1
  Trigonometric Function/1 -> Product/1
  Gain2/1 -> Trigonometric Function/1
  Motor Velocity [rad/s]/1 -> Gain2/1
  Product/1 -> Sum1/1
  Constant1/1 -> Sum1/2
  Constant6/1 -> Product/2
  Demux1/4 -> Switch4/2
  Demux1/3 -> Switch3/2
  Demux1/2 -> Switch2/2
  Switch2/1 -> Mux/2
  Switch3/1 -> Mux/3
  Switch4/1 -> Mux/4
  Switch1/1 -> Mux/1
  Demux1/1 -> Switch1/2
  Demux3/4 -> Switch4/3
  Demux3/3 -> Switch3/3
  Demux3/2 -> Switch2/3
  Demux3/1 -> Switch1/3
  Stance/Flight [1/0] x4/1 -> Demux1/1
  Constant2/1 -> Switch1/1
  Constant3/1 -> Switch2/1
  Constant4/1 -> Switch3/1
  Constant5/1 -> Switch4/1
  Sum1/1 -> Demux3/1

== system spring_measurements/Control/Actuator Control/SEA Controller (Torque)/Loaded Unloaded Switch ==
  Loaded Signal : Inport
  Loaded/Unloaded [1/0] x4 : Inport  Port=2
  Unloaded Signal : Inport  Port=3
  Demux : Demux
  Demux1 : Demux
  Demux2 : Demux
  Mux : Mux
  Switch{,1..3} (4 alike) : Switch  Criteria=u2 ~= 0
  Signal : Outport
  wires:
  Demux2/1 -> Switch/3
  Demux2/2 -> Switch1/3
  Demux2/3 -> Switch2/3
  Demux2/4 -> Switch3/3
  Unloaded Signal/1 -> Demux2/1
  Demux1/4 -> Switch3/1
  Demux1/3 -> Switch2/1
  Demux1/2 -> Switch1/1
  Demux1/1 -> Switch/1
  Loaded Signal/1 -> Demux1/1
  Demux/1 -> Switch/2
  Switch/1 -> Mux/1
  Mux/1 -> Signal/1
  Loaded/Unloaded [1/0] x4/1 -> Demux/1
  Switch3/1 -> Mux/4
  Switch2/1 -> Mux/3
  Switch1/1 -> Mux/2
  Demux/2 -> Switch1/2
  Demux/3 -> Switch2/2
  Demux/4 -> Switch3/2

== system spring_measurements/Control/Actuator Control/SEA Controller (Torque)/Stance Flight Kd Switch ==
  Kd Stance : Inport
  Stance/Flight [1/0] x4 : Inport  Port=2
  Kd Flight : Inport  Port=3
  Demux : Demux
  Demux1 : Demux
  Demux2 : Demux
  Mux : Mux
  Switch{,1..3} (4 alike) : Switch  Criteria=u2 ~= 0
  Kd : Outport
  wires:
  Demux/4 -> Switch3/2
  Demux/3 -> Switch2/2
  Demux/2 -> Switch1/2
  Switch1/1 -> Mux/2
  Switch2/1 -> Mux/3
  Switch3/1 -> Mux/4
  Stance/Flight [1/0] x4/1 -> Demux/1
  Mux/1 -> Kd/1
  Switch/1 -> Mux/1
  Demux/1 -> Switch/2
  Kd Stance/1 -> Demux1/1
  Demux1/1 -> Switch/1
  Demux1/2 -> Switch1/1
  Demux1/3 -> Switch2/1
  Demux1/4 -> Switch3/1
  Kd Flight/1 -> Demux2/1
  Demux2/4 -> Switch3/3
  Demux2/3 -> Switch2/3
  Demux2/2 -> Switch1/3
  Demux2/1 -> Switch/3

== system spring_measurements/Control/Actuator Control/SEA Controller (Torque)/Stance Flight Kp Switch ==
  Kp Stance : Inport
  Stance/Flight [1/0] x4 : Inport  Port=2
  Kp Flight : Inport  Port=3
  Demux : Demux
  Mux : Mux
  Switch{,1..3} (4 alike) : Switch  Criteria=u2 ~= 0
  Kp : Outport
  wires:
  Kp Flight/1 -> Switch/3, Switch3/3, Switch2/3, Switch1/3
  Kp Stance/1 -> Switch3/1, Switch2/1, Switch1/1, Switch/1
  Demux/1 -> Switch/2
  Switch/1 -> Mux/1
  Mux/1 -> Kp/1
  Stance/Flight [1/0] x4/1 -> Demux/1
  Switch3/1 -> Mux/4
  Switch2/1 -> Mux/3
  Switch1/1 -> Mux/2
  Demux/2 -> Switch1/2
  Demux/3 -> Switch2/2
  Demux/4 -> Switch3/2

== system spring_measurements/Control/Actuator Control/SEA Controller (Torque)/dtau_des ==
  x : Inport
  Gain1 : Gain  Gain=1/sample_time
  difference : simulink/Discrete/Difference  ICPrevInput=0.0  InputProcessing=Inherited  OutMin=[]  OutMax=[]  OutDataType=fixdt(1, 16)  OutScaling=2^-10  DoSatur=off
  two_pole_filter : DiscreteTransferFcn  Numerator=[A_lpf_dtau 0 0]  Denominator=[1 B1_lpf_dtau B2_lpf_dtau]  SampleTime=sample_time
  dx/dt : Outport
  wires:
  two_pole_filter/1 -> dx/dt/1
  x/1 -> Gain1/1
  difference/1 -> two_pole_filter/1
  Gain1/1 -> difference/1

== system spring_measurements/Control/Actuator Control/SEA Controller (Torque)/filtered_derivative ==
  x : Inport
  Gain1 : Gain  Gain=1/sample_time
  difference : simulink/Discrete/Difference  ICPrevInput=0.0  InputProcessing=Inherited  OutMin=[]  OutMax=[]  OutDataType=fixdt(1, 16)  OutScaling=2^-10  DoSatur=off
  two_pole_filter : DiscreteTransferFcn  Numerator=[A_lpf_accel 0 0]  Denominator=[1 B1_lpf_accel B2_lpf_accel]  SampleTime=sample_time
  dx/dt : Outport
  wires:
  Gain1/1 -> difference/1
  difference/1 -> two_pole_filter/1
  x/1 -> Gain1/1
  two_pole_filter/1 -> dx/dt/1

== system spring_measurements/Control/Actuator Control/SEA Controller (Torque) 1/Antiresonance Compensation ==
  Torque : Inport
  Notch Filter (Flight) : DiscreteTransferFcn  Numerator=[K_notch_f1 K_notch_f1*A1_notch_f1 K_notch_f1*A2_notch_f1]  Denominator=[1 B1_notch_f1 B2_notch_f1]  SampleTime=sample_time
  Filtered Torque : Outport
  wires:
  Notch Filter (Flight)/1 -> Filtered Torque/1
  Torque/1 -> Notch Filter (Flight)/1

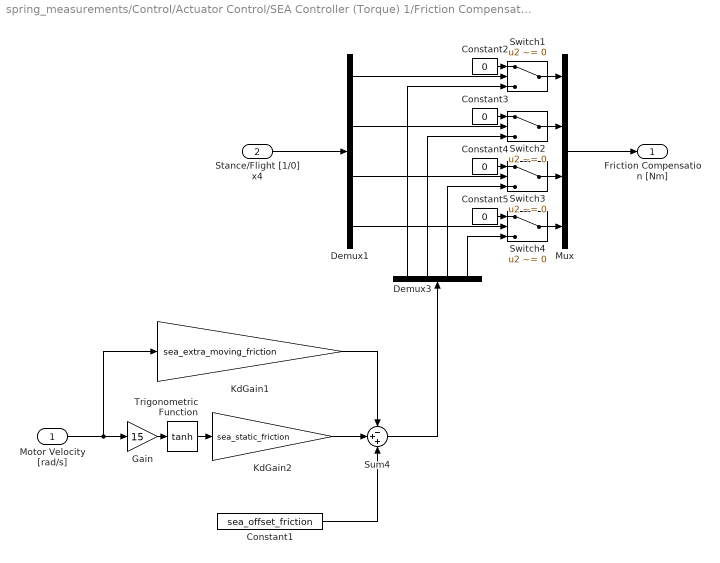
== system spring_measurements/Control/Actuator Control/SEA Controller (Torque) 1/Friction Compensation ==
  Motor Velocity [rad/s] : Inport
  Stance/Flight [1/0] x4 : Inport  Port=2
  Constant1 : Constant  Value=sea_offset_friction
  Constant{2..5} (4 alike) : Constant  Value=0
  Demux1 : Demux
  Demux3 : Demux
  Gain : Gain  Gain=15
  KdGain1 : Gain  Description=xPCTag(1)=kd_sea_torque;  Gain=sea_extra_moving_friction
  KdGain2 : Gain  Description=xPCTag(1)=kd_sea_torque;  Gain=sea_static_friction
  Mux : Mux
  Sum4 : Sum  Inputs=-++
  Switch{1..4} (4 alike) : Switch  Criteria=u2 ~= 0
  Trigonometric Function : Trigonometry  Operator=tanh
  Friction Compensation [Nm] : Outport
  wires:
  KdGain1/1 -> Sum4/1
  Constant1/1 -> Sum4/3
  KdGain2/1 -> Sum4/2
  Trigonometric Function/1 -> KdGain2/1
  Gain/1 -> Trigonometric Function/1
  Motor Velocity [rad/s]/1 -> Gain/1, KdGain1/1
  Demux1/4 -> Switch4/2
  Demux1/3 -> Switch3/2
  Demux1/2 -> Switch2/2
  Switch2/1 -> Mux/2
  Switch3/1 -> Mux/3
  Switch4/1 -> Mux/4
  Switch1/1 -> Mux/1
  Demux1/1 -> Switch1/2
  Demux3/4 -> Switch4/3
  Demux3/3 -> Switch3/3
  Demux3/2 -> Switch2/3
  Demux3/1 -> Switch1/3
  Stance/Flight [1/0] x4/1 -> Demux1/1
  Constant2/1 -> Switch1/1
  Constant3/1 -> Switch2/1
  Constant4/1 -> Switch3/1
  Constant5/1 -> Switch4/1
  Sum4/1 -> Demux3/1
  Mux/1 -> Friction Compensation [Nm]/1

== system spring_measurements/Control/Actuator Control/SEA Controller (Torque) 1/Loaded Unloaded Switch ==
  Loaded Signal : Inport
  Loaded/Unloaded [1/0] x4 : Inport  Port=2
  Unloaded Signal : Inport  Port=3
  Demux : Demux
  Demux1 : Demux
  Demux2 : Demux
  Mux : Mux
  Switch{,1..3} (4 alike) : Switch  Criteria=u2 ~= 0
  Signal : Outport
  wires:
  Demux2/1 -> Switch/3
  Demux2/2 -> Switch1/3
  Demux2/3 -> Switch2/3
  Demux2/4 -> Switch3/3
  Unloaded Signal/1 -> Demux2/1
  Demux1/4 -> Switch3/1
  Demux1/3 -> Switch2/1
  Demux1/2 -> Switch1/1
  Demux1/1 -> Switch/1
  Loaded Signal/1 -> Demux1/1
  Demux/1 -> Switch/2
  Switch/1 -> Mux/1
  Mux/1 -> Signal/1
  Loaded/Unloaded [1/0] x4/1 -> Demux/1
  Switch3/1 -> Mux/4
  Switch2/1 -> Mux/3
  Switch1/1 -> Mux/2
  Demux/2 -> Switch1/2
  Demux/3 -> Switch2/2
  Demux/4 -> Switch3/2

== system spring_measurements/Control/Actuator Control/SEA Controller (Torque) 1/Stance Flight Kd Switch ==
  Kd Stance : Inport
  Stance/Flight [1/0] x4 : Inport  Port=2
  Kd Flight : Inport  Port=3
  Demux : Demux
  Demux1 : Demux
  Demux2 : Demux
  Mux : Mux
  Switch{,1..3} (4 alike) : Switch  Criteria=u2 ~= 0
  Kd : Outport
  wires:
  Demux/4 -> Switch3/2
  Demux/3 -> Switch2/2
  Demux/2 -> Switch1/2
  Switch1/1 -> Mux/2
  Switch2/1 -> Mux/3
  Switch3/1 -> Mux/4
  Stance/Flight [1/0] x4/1 -> Demux/1
  Mux/1 -> Kd/1
  Switch/1 -> Mux/1
  Demux/1 -> Switch/2
  Kd Stance/1 -> Demux1/1
  Demux1/1 -> Switch/1
  Demux1/2 -> Switch1/1
  Demux1/3 -> Switch2/1
  Demux1/4 -> Switch3/1
  Kd Flight/1 -> Demux2/1
  Demux2/4 -> Switch3/3
  Demux2/3 -> Switch2/3
  Demux2/2 -> Switch1/3
  Demux2/1 -> Switch/3

== system spring_measurements/Control/Actuator Control/SEA Controller (Torque) 1/Stance Flight Kp Switch ==
  Kp Stance : Inport
  Stance/Flight [1/0] x4 : Inport  Port=2
  Kp Flight : Inport  Port=3
  Demux : Demux
  Mux : Mux
  Switch{,1..3} (4 alike) : Switch  Criteria=u2 ~= 0
  Kp : Outport
  wires:
  Kp Flight/1 -> Switch/3, Switch3/3, Switch2/3, Switch1/3
  Kp Stance/1 -> Switch3/1, Switch2/1, Switch1/1, Switch/1
  Demux/1 -> Switch/2
  Switch/1 -> Mux/1
  Mux/1 -> Kp/1
  Stance/Flight [1/0] x4/1 -> Demux/1
  Switch3/1 -> Mux/4
  Switch2/1 -> Mux/3
  Switch1/1 -> Mux/2
  Demux/2 -> Switch1/2
  Demux/3 -> Switch2/2
  Demux/4 -> Switch3/2

== system spring_measurements/Control/Actuator Control/SEA Controller (Torque) 1/dtau_des ==
  x : Inport
  Gain1 : Gain  Gain=1/sample_time
  difference : simulink/Discrete/Difference  ICPrevInput=0.0  InputProcessing=Inherited  OutMin=[]  OutMax=[]  OutDataType=fixdt(1, 16)  OutScaling=2^-10  DoSatur=off
  two_pole_filter : DiscreteTransferFcn  Numerator=[A_lpf_dtau 0 0]  Denominator=[1 B1_lpf_dtau B2_lpf_dtau]  SampleTime=sample_time
  dx/dt : Outport
  wires:
  two_pole_filter/1 -> dx/dt/1
  x/1 -> Gain1/1
  difference/1 -> two_pole_filter/1
  Gain1/1 -> difference/1

== system spring_measurements/Control/Actuator Control/SEA Controller (Torque) 1/filtered_derivative ==
  x : Inport
  Gain1 : Gain  Gain=1/sample_time
  difference : simulink/Discrete/Difference  ICPrevInput=0.0  InputProcessing=Inherited  OutMin=[]  OutMax=[]  OutDataType=fixdt(1, 16)  OutScaling=2^-10  DoSatur=off
  two_pole_filter : DiscreteTransferFcn  Numerator=[A_lpf_accel 0 0]  Denominator=[1 B1_lpf_accel B2_lpf_accel]  SampleTime=sample_time
  dx/dt : Outport
  wires:
  Gain1/1 -> difference/1
  difference/1 -> two_pole_filter/1
  x/1 -> Gain1/1
  two_pole_filter/1 -> dx/dt/1

== system spring_measurements/Control/Behavior Control/lateral_PID_control/Lateral Hip PID ==
  position_error : Inport
  velocity_error : Inport  Port=2
  Discrete-Time Integrator : DiscreteIntegrator  IntegratorMethod=Integration: Trapezoidal  SampleTime=sample_time  LimitOutput=on  UpperSaturationLimit=i_limit_lateral  LowerSaturationLimit=-i_limit_lateral  ICPrevOutput=DiscIntNeverNeededParam  ICPrevScaledInput=DiscIntNeverNeededParam
  Proportional Gain : Gain  Description=xPCTag(1)=kp_lateral;  Gain=kp_lateral
  Proportional Gain1 : Gain  Description=xPCTag(1)=kd_lateral;  Gain=kd_lateral
  Proportional Gain2 : Gain  Description=xPCTag(1)=ki_lateral;  Gain=ki_lateral
  Sum : Sum  Inputs=+++
  out : Outport
  wires:
  Proportional Gain1/1 -> Sum/1
  Sum/1 -> out/1
  position_error/1 -> Proportional Gain/1, Proportional Gain2/1
  Proportional Gain/1 -> Sum/2
  Proportional Gain2/1 -> Discrete-Time Integrator/1
  Discrete-Time Integrator/1 -> Sum/3
  velocity_error/1 -> Proportional Gain1/1

== system spring_measurements/Control/Behavior Control/lateral_PID_control/spherical_correction_angle ==
  q_cmu : Inport
  Selector : Selector  InputPortWidth=13  Indices=[11]
  Sum1 : Sum  Inputs=|+-
  Terminator2 : Terminator
  boom_mount_angle : Constant  Value=boom_mount_angle
  lateral_correction : Gain  Gain=180/pi
  lateral_correction [rad] : Outport
  wires:
  lateral_correction/1 -> Terminator2/1
  boom_mount_angle/1 -> Sum1/2
  q_cmu/1 -> Selector/1
  Selector/1 -> Sum1/1  "qBoomRoll"
  Sum1/1 -> lateral_correction [rad]/1, lateral_correction/1
